simulink model "Robot_leg_3"  (R2018a)
settings: Solver=VariableStepAuto  StartTime=0.0  StopTime=10  RelTol=1e-3
model workspace: external: MATLAB File E:\Humanoid\Simscape model\Simscape_model_2\simscape_model\Robot_leg_2_DataFile.m (data not in the file)
values from neighbouring files (symbols this model uses):
  m = 0    [Trajectory_generation_initial.m]    (also in final_gait.m)
undefined symbols (not defined in the file or in its folder): height_plane, smiData, X, Y, Z
libraries: sm_lib x69, nesl_utility x52, simulink x49, walkingRobotUtils x14, Contact_Forces_Lib x8
(part 1 of 3)
settings Model: SimulationMode=external  Creator=Workstation-1  LastModifiedBy=Workstation-1
settings GRTTargetCC: ExtMode=on
settings DiagnosticsConfigSet: SimMechanicsRigidlyBoundBlock=none

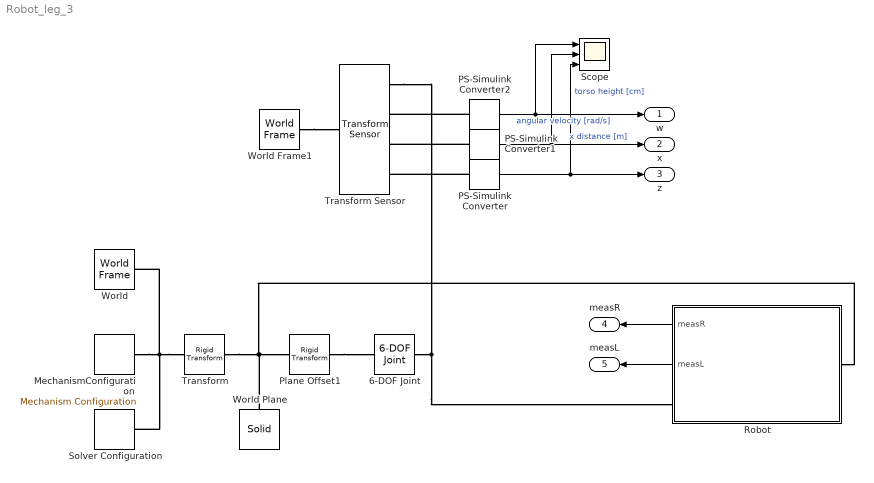
== system Robot_leg_3 ==
  6-DOF Joint : sm_lib/Joints/6-DOF Joint  SenseConstraintForce=off  SenseConstraintForceX=off  SenseConstraintForceY=off  SenseConstraintForceZ=off  SenseConstraintTorque=off  SenseConstraintTorqueX=off  SenseConstraintTorqueY=off  SenseConstraintTorqueZ=off  SenseTotalForce=off  SenseTotalForceX=off  SenseTotalForceY=off  SenseTotalForceZ=off  SenseTotalTorque=off  SenseTotalTorqueX=off  SenseTotalTorqueY=off  SenseTotalTorqueZ=off  CompositeWrenchDir=FollowerOnBase  CompositeWrenchFrame=BaseFrame  PxEquilibriumPosition=0  PxEquilibriumPositionUnits=m  PxSpringStiffness=0  PxSpringStiffnessUnits=N/m  PxDampingCoefficient=world_damping  PxDampingCoefficientUnits=N/(m/s)  PxTorqueActuationMode=NoTorque  PxMotionActuationMode=ComputedMotion  PxSensePosition=off  PxSenseVelocity=off  PxSenseAcceleration=off  PxSenseTorqueForce=off  PxPositionTargetSpecify=on  PxPositionTargetPriority=High  PxPositionTargetValue=0  PxPositionTargetValueUnits=m  PxVelocityTargetSpecify=off  PxVelocityTargetPriority=High  PxVelocityTargetValue=0  PxVelocityTargetValueUnits=m/s  PyEquilibriumPosition=0  PyEquilibriumPositionUnits=m  PySpringStiffness=0  PySpringStiffnessUnits=N/m  PyDampingCoefficient=world_damping  PyDampingCoefficientUnits=N/(m/s)  PyTorqueActuationMode=NoTorque  PyMotionActuationMode=ComputedMotion  PySensePosition=off  PySenseVelocity=off  PySenseAcceleration=off  PySenseTorqueForce=off  PyPositionTargetSpecify=on  PyPositionTargetPriority=High  PyPositionTargetValue=0  PyPositionTargetValueUnits=m  PyVelocityTargetSpecify=off  PyVelocityTargetPriority=High  PyVelocityTargetValue=0  PyVelocityTargetValueUnits=m/s  PzEquilibriumPosition=0  PzEquilibriumPositionUnits=m  PzSpringStiffness=0  PzSpringStiffnessUnits=N/m  PzDampingCoefficient=world_damping  PzDampingCoefficientUnits=N/(m/s)  PzTorqueActuationMode=NoTorque  PzMotionActuationMode=ComputedMotion  PzSensePosition=off  PzSenseVelocity=off  PzSenseAcceleration=off  PzSenseTorqueForce=off  PzPositionTargetSpecify=on  PzPositionTargetPriority=High  PzPositionTargetValue=init_height  PzPositionTargetValueUnits=cm  PzVelocityTargetSpecify=off  PzVelocityTargetPriority=High  PzVelocityTargetValue=0  PzVelocityTargetValueUnits=m/s  SphDefPosRotationMethod=None  SphDefPosRotationAngleUnits=deg  SphDefPosRotationStandardAxis=+Z  SphDefPosRotationAngle=0.0  SphDefPosRotationArbitraryAxis=[0 0 1]  SphDefPosFollAlignAxisA=+X  SphDefPosBaseAlignAxisA=+Y  SphDefPosFollAlignAxisB=+Y  SphDefPosBaseAlignAxisB=+Z  SphDefPosRotationSequenceAxes=FollowerAxes  SphDefPosRotationSequence=XYX  SphDefPosRotationSequenceAngles=[0 0 0]  SphDefPosRotationSequenceAnglesUnits=deg  SphDefPosRotationMatrix=[1 0 0; 0 1 0; 0 0 1]  SphEqPosRotationMethod=None  SphEqPosRotationAngleUnits=deg  SphEqPosRotationStandardAxis=+Z  SphEqPosRotationAngle=0.0  SphEqPosRotationArbitraryAxis=[0 0 1]  SphEqPosFollAlignAxisA=+X  SphEqPosBaseAlignAxisA=+Y  SphEqPosFollAlignAxisB=+Y  SphEqPosBaseAlignAxisB=+Z  SphEqPosRotationSequenceAxes=FollowerAxes  SphEqPosRotationSequence=XYX  SphEqPosRotationSequenceAngles=[0 0 0]  SphEqPosRotationSequenceAnglesUnits=deg  SphEqPosRotationMatrix=[1 0 0; 0 1 0; 0 0 1]  SphSpringStiffness=0  SphSpringStiffnessUnits=N*m/deg  SphDampingCoefficient=world_rot_damping  SphDampingCoefficientUnits=N*m/(rad/s)  SphActuateTorqueX=off  SphActuateTorqueY=off  SphActuateTorqueZ=off  SphActuateTorque=off  SphTorqueActuationMode=NoTorque  SphMotionActuationMode=ComputedMotion  SphActuationFrame=BaseFrame  SphSensePosition=off  SphSenseVelocityX=off  SphSenseVelocityY=off  SphSenseVelocityZ=off  SphSenseVelocity=off  SphSenseAccelerationX=off  SphSenseAccelerationY=off  SphSenseAccelerationZ=off  SphSenseAcceleration=off  SphSenseTorqueX=off  SphSenseTorqueY=off  SphSenseTorqueZ=off  SphSenseTorqueForce=off  SphSensingFrame=BaseFrame  SphPositionTargetRotationMethod=None  SphPositionTargetRotationAngleUnits=deg  SphPositionTargetRotationStandardAxis=+Z  SphPositionTargetRotationAngle=0.0  SphPositionTargetRotationArbitraryAxis=[0 0 1]  SphPositionTargetFollAlignAxisA=+X  SphPositionTargetBaseAlignAxisA=+Y  SphPositionTargetFollAlignAxisB=+Y  SphPositionTargetBaseAlignAxisB=+Z  SphPositionTargetRotationSequenceAxes=FollowerAxes  SphPositionTargetRotationSequence=XYX  SphPositionTargetRotationSequenceAngles=[0 0 0]  SphPositionTargetRotationSequenceAnglesUnits=deg  SphPositionTargetRotationMatrix=eye(3)  SphPositionTargetSpecify=off  SphPositionTargetPriority=High  SphVelocityTargetValue=[0 0 0]  SphVelocityTargetValueUnits=deg/s  SphVelocityTargetSpecify=off  SphVelocityTargetPriority=High  SphVelocityTargetInFollowerFrame=on
  MechanismConfiguration : sm_lib/Utilities/Mechanism Configuration  UniformGravity=Constant  GravityVector=[0 0 -9.80665]  GravityUnits=m/s^2  LinearizationDelta=0.001
  PS-Simulink Converter : nesl_utility/PS-Simulink Converter  PhysicalDomain=network_engine_domain  SubClassName=ps_output  LeftPortType=input  RightPortType=output  PseudoPeriodic=off  Frequencies=[]  Unit=cm  AffineConversion=off
  PS-Simulink Converter1 : nesl_utility/PS-Simulink Converter  PhysicalDomain=network_engine_domain  SubClassName=ps_output  LeftPortType=input  RightPortType=output  PseudoPeriodic=off  Frequencies=[]  Unit=m  AffineConversion=off
  PS-Simulink Converter2 : nesl_utility/PS-Simulink Converter  PhysicalDomain=network_engine_domain  SubClassName=ps_output  LeftPortType=input  RightPortType=output  PseudoPeriodic=off  Frequencies=[]  Unit=rad/s  AffineConversion=off
  Plane Offset1 : sm_lib/Frames and Transforms/Rigid Transform  TranslationMethod=StandardAxis  TranslationStandardOffset=height_plane/2  TranslationLengthUnit=m  TranslationStandardAxis=+Z  TranslationCartesianOffset=[0 0 0]  TranslationROffset=0  TranslationROffsetUnits=m  TranslationZOffset=0  TranslationZOffsetUnits=m  TranslationThetaOffset=0  TranslationThetaOffsetUnits=deg  RotationMethod=None  RotationAngleUnits=deg  RotationStandardAxis=+Z  RotationAngle=0.0  RotationArbitraryAxis=[0 0 1]  FollAlignAxisA=+X  BaseAlignAxisA=+Y  FollAlignAxisB=+Y  BaseAlignAxisB=+Z  RotationSequenceAxes=FollowerAxes  RotationSequence=XYX  RotationSequenceAngles=[0 0 0]  RotationSequenceAnglesUnits=deg  RotationMatrix=[1 0 0; 0 1 0; 0 0 1]
  Robot : Subsystem
  Scope : Scope  NumInputPorts=3
  Solver Configuration : nesl_utility/Solver Configuration  PhysicalDomain=network_engine_domain  SubClassName=solver  LeftPortType=input  RightPortType=generic  Tones=[]  Harmonics=[]  SimulateNoise=off  Profile=off  UseLocalSampling=off  EnableSwitchedLinearOptims=on  FrequencyDomain=off  UseCCode=off  RelTol=0.001  AbsTol=1e-06  MinStep=1e-09  ToWorkspace=off  RevertToSquareIcSolve=off  NumHomotopyIterations=100  PhasorMode=off  PhasorModeNumHarmonics=1  DoDC=off  ResidualTolerance=1e-09  UseLocalSolver=off  LocalSolverChoice=NE_BACKWARD_EULER_ADVANCER  LocalSolverSampleTime=0.001  DoFixedCost=off  MaxNonlinIter=3  MaxModeIter=2  LinearAlgebra=Sparse  EquationFormulation=NE_TIME_EF  DelaysMemoryBudget=1024  AutomaticFiltering=on  FilteringTimeConstant=0.001
  Transform : sm_lib/Frames and Transforms/Rigid Transform  TranslationMethod=Cartesian  TranslationStandardOffset=0  TranslationLengthUnit=mm  TranslationStandardAxis=+Z  TranslationCartesianOffset=smiData.RigidTransform(22).translation  TranslationROffset=0  TranslationROffsetUnits=m  TranslationZOffset=0  TranslationZOffsetUnits=m  TranslationThetaOffset=0  TranslationThetaOffsetUnits=deg  RotationMethod=ArbitraryAxis  RotationAngleUnits=rad  RotationStandardAxis=+Z  RotationAngle=smiData.RigidTransform(22).angle  RotationArbitraryAxis=smiData.RigidTransform(22).axis  FollAlignAxisA=+X  BaseAlignAxisA=+Y  FollAlignAxisB=+Y  BaseAlignAxisB=+Z  RotationSequenceAxes=FollowerAxes  RotationSequence=XYX  RotationSequenceAngles=[0 0 0]  RotationSequenceAnglesUnits=deg  RotationMatrix=[1 0 0; 0 1 0; 0 0 1]
  Transform Sensor : sm_lib/Frames and Transforms/Transform Sensor  MeasurementFrame=World  SenseAngle=off  SenseAxis=off  SenseAngle1=off  SenseAngle2=off  SenseAngle3=off  SenseQ=off  SenseR=off  SenseOmegaX=off  SenseOmegaY=off  SenseOmegaZ=on  SenseOmega1=off  SenseOmega2=off  SenseOmega3=off  SenseQDot=off  SenseRDot=off  SenseAlphaX=off  SenseAlphaY=off  SenseAlphaZ=off  SenseAlpha1=off  SenseAlpha2=off  SenseAlpha3=off  SenseQDDot=off  SenseRDDot=off  SenseX=on  SenseY=off  SenseZ=on  SenseRad=off  SenseAzim=off  SenseDist=off  SenseInc=off  SenseXDot=off  SenseYDot=off  SenseZDot=off  SenseRadDot=off  SenseAzimDot=off  SenseDistDot=off  SenseIncDot=off  SenseXDDot=off  SenseYDDot=off  SenseZDDot=off  SenseRadDDot=off  SenseAzimDDot=off  SenseDistDDot=off  SenseIncDDot=off
  World : sm_lib/Frames and Transforms/World Frame
  World Frame1 : sm_lib/Frames and Transforms/World Frame
  World Plane : sm_lib/Body Elements/Solid  InertiaType=CalculateFromGeometry  Mass=1  MassUnits=kg  CenterOfMass=[0 0 0]  CenterOfMassUnits=m  MomentsOfInertia=[1 1 1]  MomentsOfInertiaUnits=kg*m^2  ProductsOfInertia=[0 0 0]  ProductsOfInertiaUnits=kg*m^2  DensityBased=on  Density=density  DensityUnits=kg/(m^3)  DoExposeReferenceFrame=on  SerializedFrames=<Frames/>  GraphicType=FromGeometry  MarkerShape=Sphere  MarkerSize=10  MarkerSizeUnits=m  GraphicVisPropType=SimpleVisualProperties  GraphicDiffuseColor=[1.0 1.0 0.8]  GraphicSpecularColor=[0.5 0.5 0.5 1.0]  GraphicAmbientColor=[0.15 0.15 0.15 1.0]  GraphicEmissiveColor=[0.0 0.0 0.0 1.0]  GraphicShininess=75  GraphicOpacity=0.5  GeometryShape=Brick  RectangleSize=[1 1]  RectangleSizeUnits=m  BrickDimensions="[10 3  0.025]"  BrickDimensionUnits=m  CylinderRadius=1  CylinderRadiusUnits=m  CylinderLength=1  CylinderLengthUnits=m  SphereRadius=1  SphereRadiusUnits=m  EllipsoidRadii=[1 1 1]  EllipsoidRadiiUnits=m  ExtrusionCrossSection=[1 1; -1 1; -1 -1; 1 -1]  ExtrusionCrossSectionUnits=m  ExtrusionLength=1  ExtrusionLengthUnits=m  PolygonNumSides=3  PolygonOuterRadius=1  PolygonOuterRadiusUnits=m  ExtGeomFileType=STL  ExtGeomFileUnits=m  RevolutionCrossSection=[1 1; 1 -1; 2 -1; 2 1]  RevolutionCrossSectionUnits=m  RevolutionExtent=Full  RevolutionAngle=180  RevolutionAngleUnits=deg
  w : Outport
  x : Outport  Port=2
  z : Outport  Port=3
  measR : Outport  Port=4
  measL : Outport  Port=5
  wires:
  PS-Simulink Converter/1 -> Scope/3, z/1  "torso height [cm]"
  PS-Simulink Converter2/1 -> Scope/1, w/1  "angular velocity [rad/s]"
  PS-Simulink Converter1/1 -> Scope/2, x/1  "x distance [m]"
  Robot/1(measR) -> measR/1
  Robot/2(measL) -> measL/1
  connections:
  Transform/LConn1 -- Solver Configuration/RConn1 -- MechanismConfiguration/RConn1 -- World/RConn1
  Transform/RConn1 -- Plane Offset1/LConn1 -- World Plane/RConn1 -- Robot/LConn1
  6-DOF Joint/RConn1 -- Robot/RConn1 -- Transform Sensor/RConn1
  Plane Offset1/RConn1 -- 6-DOF Joint/LConn1
  PS-Simulink Converter1/LConn1 -- Transform Sensor/RConn3
  PS-Simulink Converter/LConn1 -- Transform Sensor/RConn4
  PS-Simulink Converter2/LConn1 -- Transform Sensor/RConn2
  World Frame1/RConn1 -- Transform Sensor/LConn1

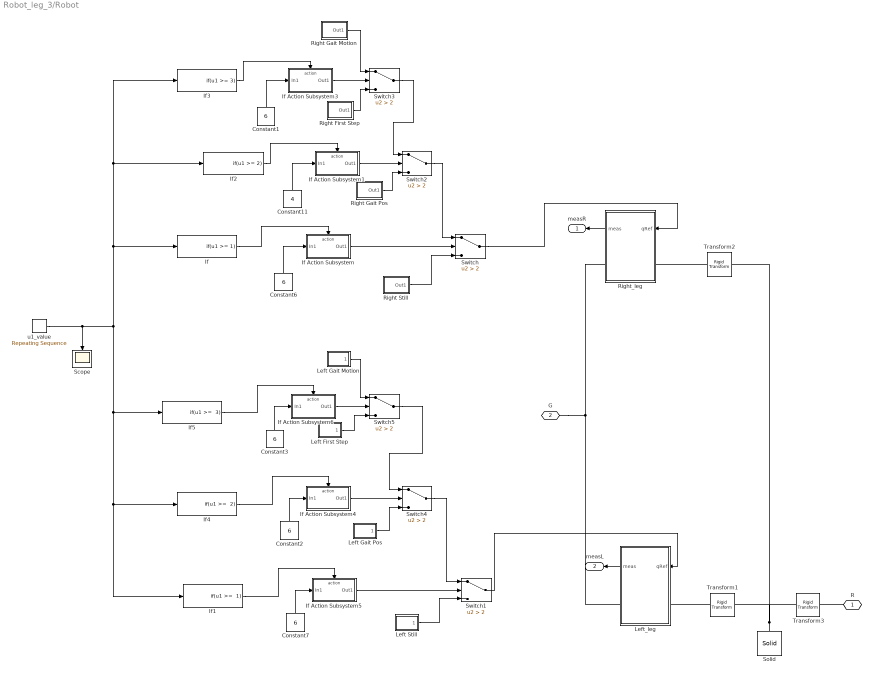
== system Robot_leg_3/Robot ==
  Constant{1..3,6..7} (5 alike) : Constant  Value=6
  Constant11 : Constant  Value=4
  If : If  IfExpression=u1 >= 1  ShowElse=off
  If Action Subsystem : Subsystem  TreatAsAtomicUnit=on
  If Action Subsystem1 : Subsystem  TreatAsAtomicUnit=on
  If Action Subsystem3 : Subsystem  TreatAsAtomicUnit=on
  If Action Subsystem4 : Subsystem  TreatAsAtomicUnit=on
  If Action Subsystem5 : Subsystem  TreatAsAtomicUnit=on
  If Action Subsystem6 : Subsystem  TreatAsAtomicUnit=on
  If1 : If  IfExpression="u1 >=  1"  ShowElse=off
  If2 : If  IfExpression=u1 >= 2  ShowElse=off
  If3 : If  IfExpression=u1 >= 3  ShowElse=off
  If4 : If  IfExpression="u1 >=  2"  ShowElse=off
  If5 : If  IfExpression="u1 >=  3"  ShowElse=off
  Left First Step : Subsystem
  Left Gait Motion : Subsystem
  Left Gait Pos : Subsystem
  Left Still : Subsystem
  Left_leg : Subsystem
  Right First Step : Subsystem
  Right Gait Motion : Subsystem
  Right Gait Pos : Subsystem
  Right Still : Subsystem
  Right_leg : Subsystem
  Scope : Scope
  Solid : sm_lib/Body Elements/Solid  InertiaType=Custom  Mass=smiData.Solid(13).mass  MassUnits=kg  CenterOfMass=smiData.Solid(13).CoM  CenterOfMassUnits=mm  MomentsOfInertia=smiData.Solid(13).MoI  MomentsOfInertiaUnits=kg*mm^2  ProductsOfInertia=smiData.Solid(13).PoI  ProductsOfInertiaUnits=kg*mm^2  DensityBased=on  Density=1000  DensityUnits=kg/m^3  DoExposeReferenceFrame=on  SerializedFrames=<Frames/>  GraphicType=FromGeometry  MarkerShape=Sphere  MarkerSize=10  GraphicVisPropType=SimpleVisualProperties  GraphicDiffuseColor=smiData.Solid(13).color  GraphicSpecularColor=[0.5 0.5 0.5 1.0]  GraphicAmbientColor=[0.15 0.15 0.15 1.0]  GraphicEmissiveColor=[0.0 0.0 0.0 1.0]  GraphicShininess=75  GraphicOpacity=smiData.Solid(13).opacity  GeometryShape=FromFile  RectangleSize=[1 1]  RectangleSizeUnits=m  BrickDimensions=[1 1 1]  BrickDimensionUnits=m  CylinderRadius=1  CylinderRadiusUnits=m  CylinderLength=1  CylinderLengthUnits=m  SphereRadius=1  SphereRadiusUnits=m  EllipsoidRadii=[1 1 1]  EllipsoidRadiiUnits=m  ExtrusionCrossSection=[1 1; -1 1; -1 -1; 1 -1]  ExtrusionCrossSectionUnits=m  ExtrusionLength=1  ExtrusionLengthUnits=m  PolygonNumSides=3  PolygonOuterRadius=1  PolygonOuterRadiusUnits=m  ExtGeomFileType=STEP  ExtGeomFileName=Torso_Default_sldprt.STEP  ExtGeomFileUnits=m  RevolutionCrossSection=[1 1; 1 -1; 2 -1; 2 1]  RevolutionCrossSectionUnits=m  RevolutionExtent=Full  RevolutionAngle=180  RevolutionAngleUnits=deg
  Switch{,1..5} (6 alike) : Switch  Criteria=u2 > Threshold  Threshold=2
  Transform1 : sm_lib/Frames and Transforms/Rigid Transform  TranslationMethod=Cartesian  TranslationStandardOffset=0  TranslationLengthUnit=mm  TranslationStandardAxis=+Z  TranslationCartesianOffset=smiData.RigidTransform(17).translation  TranslationROffset=0  TranslationROffsetUnits=m  TranslationZOffset=0  TranslationZOffsetUnits=m  TranslationThetaOffset=0  TranslationThetaOffsetUnits=deg  RotationMethod=ArbitraryAxis  RotationAngleUnits=rad  RotationStandardAxis=+Z  RotationAngle=smiData.RigidTransform(17).angle  RotationArbitraryAxis=smiData.RigidTransform(17).axis  FollAlignAxisA=+X  BaseAlignAxisA=+Y  FollAlignAxisB=+Y  BaseAlignAxisB=+Z  RotationSequenceAxes=FollowerAxes  RotationSequence=XYX  RotationSequenceAngles=[0 0 0]  RotationSequenceAnglesUnits=deg  RotationMatrix=[1 0 0; 0 1 0; 0 0 1]
  Transform2 : sm_lib/Frames and Transforms/Rigid Transform  TranslationMethod=Cartesian  TranslationStandardOffset=0  TranslationLengthUnit=mm  TranslationStandardAxis=+Z  TranslationCartesianOffset=smiData.RigidTransform(19).translation  TranslationROffset=0  TranslationROffsetUnits=m  TranslationZOffset=0  TranslationZOffsetUnits=m  TranslationThetaOffset=0  TranslationThetaOffsetUnits=deg  RotationMethod=ArbitraryAxis  RotationAngleUnits=rad  RotationStandardAxis=+Z  RotationAngle=smiData.RigidTransform(19).angle  RotationArbitraryAxis=smiData.RigidTransform(19).axis  FollAlignAxisA=+X  BaseAlignAxisA=+Y  FollAlignAxisB=+Y  BaseAlignAxisB=+Z  RotationSequenceAxes=FollowerAxes  RotationSequence=XYX  RotationSequenceAngles=[0 0 0]  RotationSequenceAnglesUnits=deg  RotationMatrix=[1 0 0; 0 1 0; 0 0 1]
  Transform3 : sm_lib/Frames and Transforms/Rigid Transform  TranslationMethod=Cartesian  TranslationStandardOffset=0  TranslationLengthUnit=mm  TranslationStandardAxis=+Z  TranslationCartesianOffset=smiData.RigidTransform(21).translation  TranslationROffset=0  TranslationROffsetUnits=m  TranslationZOffset=0  TranslationZOffsetUnits=m  TranslationThetaOffset=0  TranslationThetaOffsetUnits=deg  RotationMethod=ArbitraryAxis  RotationAngleUnits=rad  RotationStandardAxis=+Z  RotationAngle=smiData.RigidTransform(21).angle  RotationArbitraryAxis=smiData.RigidTransform(21).axis  FollAlignAxisA=+X  BaseAlignAxisA=+Y  FollAlignAxisB=+Y  BaseAlignAxisB=+Z  RotationSequenceAxes=FollowerAxes  RotationSequence=XYX  RotationSequenceAngles=[0 0 0]  RotationSequenceAnglesUnits=deg  RotationMatrix=[1 0 0; 0 1 0; 0 0 1]
  "u1_value " : simulink/Sources/Repeating Sequence  rep_seq_t=total_time  rep_seq_y=u1
  R : PMIOPort  Side=Right
  G : PMIOPort  Port=2  Side=Left
  measR : Outport
  measL : Outport  Port=2
  wires:
  "u1_value "/1 -> Scope/1, If5/1, If4/1, If1/1, If2/1, If3/1, If/1
  Switch2/1 -> Switch/1
  If1/1 -> If Action Subsystem5/Action
  Constant1/1 -> If Action Subsystem3/1(In1)
  Switch5/1 -> Switch4/1
  If/1 -> If Action Subsystem/Action
  Constant6/1 -> If Action Subsystem/1(In1)
  If Action Subsystem/1(Out1) -> Switch/2
  If Action Subsystem6/1(Out1) -> Switch5/2
  Constant7/1 -> If Action Subsystem5/1(In1)
  Constant2/1 -> If Action Subsystem4/1(In1)
  If5/1 -> If Action Subsystem6/Action
  If4/1 -> If Action Subsystem4/Action
  If Action Subsystem3/1(Out1) -> Switch3/2
  If Action Subsystem5/1(Out1) -> Switch1/2
  Switch4/1 -> Switch1/1
  Constant3/1 -> If Action Subsystem6/1(In1)
  Switch1/1 -> Left_leg/1(qRef)
  If3/1 -> If Action Subsystem3/Action
  If Action Subsystem1/1(Out1) -> Switch2/2
  Right Still/1(Out1) -> Switch/3
  Left Still/1(Out1) -> Switch1/3
  Switch3/1 -> Switch2/1
  Switch/1 -> Right_leg/1(qRef)
  If Action Subsystem4/1(Out1) -> Switch4/2
  If2/1 -> If Action Subsystem1/Action
  Constant11/1 -> If Action Subsystem1/1(In1)
  Right Gait Motion/1(Out1) -> Switch3/1
  Left Gait Motion/1(Out1) -> Switch5/1
  Left Gait Pos/1(Out1) -> Switch4/3
  Left First Step/1(Out1) -> Switch5/3
  Right First Step/1(Out1) -> Switch3/3
  Right Gait Pos/1(Out1) -> Switch2/3
  Left_leg/1(meas) -> measL/1
  Right_leg/1(meas) -> measR/1
  connections:
  Solid/RConn1 -- Transform2/LConn1 -- Transform1/LConn1 -- Transform3/LConn1
  R/RConn1 -- Transform3/RConn1
  Transform2/RConn1 -- Right_leg/LConn1
  Transform1/RConn1 -- Left_leg/LConn1
  Left_leg/RConn1 -- G/RConn1 -- Right_leg/RConn1

== system Robot_leg_3/Robot/If Action Subsystem ==
  In1 : Inport
  Action Port : ActionPort  ActionType=then
  Out1 : Outport
  wires:
  In1/1 -> Out1/1

== system Robot_leg_3/Robot/If Action Subsystem1 ==
  In1 : Inport
  Action Port : ActionPort  ActionType=then
  Out1 : Outport
  wires:
  In1/1 -> Out1/1

== system Robot_leg_3/Robot/If Action Subsystem3 ==
  In1 : Inport
  Action Port : ActionPort  ActionType=then
  Out1 : Outport
  wires:
  In1/1 -> Out1/1

== system Robot_leg_3/Robot/If Action Subsystem4 ==
  In1 : Inport
  Action Port : ActionPort  ActionType=then
  Out1 : Outport
  wires:
  In1/1 -> Out1/1

== system Robot_leg_3/Robot/If Action Subsystem5 ==
  In1 : Inport
  Action Port : ActionPort  ActionType=then
  Out1 : Outport
  wires:
  In1/1 -> Out1/1

== system Robot_leg_3/Robot/If Action Subsystem6 ==
  In1 : Inport
  Action Port : ActionPort  ActionType=then
  Out1 : Outport
  wires:
  In1/1 -> Out1/1

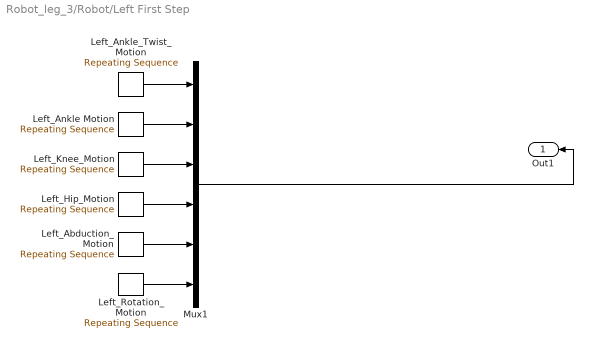
== system Robot_leg_3/Robot/Left First Step ==
  Left_Abduction_Motion : simulink/Sources/Repeating Sequence  rep_seq_t=time  rep_seq_y=left_theta_first_5
  Left_Ankle Motion : simulink/Sources/Repeating Sequence  rep_seq_t=time_first  rep_seq_y=left_theta_first_3
  Left_Ankle_Twist_Motion : simulink/Sources/Repeating Sequence  rep_seq_t=time  rep_seq_y=left_theta_first_4
  Left_Hip_Motion : simulink/Sources/Repeating Sequence  rep_seq_t=time_first  rep_seq_y=left_theta_first_1
  Left_Knee_Motion : simulink/Sources/Repeating Sequence  rep_seq_t=time_first  rep_seq_y=left_theta_first_2
  Left_Rotation_Motion : simulink/Sources/Repeating Sequence  rep_seq_t=time_first  rep_seq_y=left_theta_first_6
  Mux1 : Mux  Inputs=6
  Out1 : Outport
  wires:
  Left_Knee_Motion/1 -> Mux1/3
  Left_Rotation_Motion/1 -> Mux1/6
  Left_Hip_Motion/1 -> Mux1/4
  Left_Abduction_Motion/1 -> Mux1/5
  Left_Ankle_Twist_Motion/1 -> Mux1/1
  Left_Ankle Motion/1 -> Mux1/2
  Mux1/1 -> Out1/1

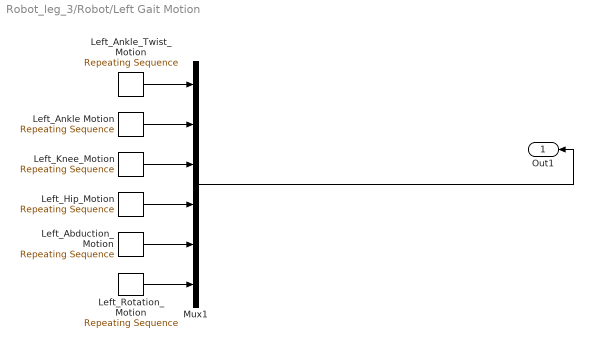
== system Robot_leg_3/Robot/Left Gait Motion ==
  Left_Abduction_Motion : simulink/Sources/Repeating Sequence  rep_seq_t=time  rep_seq_y=left_theta_5
  Left_Ankle Motion : simulink/Sources/Repeating Sequence  rep_seq_t=time  rep_seq_y=left_theta_3
  Left_Ankle_Twist_Motion : simulink/Sources/Repeating Sequence  rep_seq_t=time  rep_seq_y=left_theta_4
  Left_Hip_Motion : simulink/Sources/Repeating Sequence  rep_seq_t=time  rep_seq_y=left_theta_1
  Left_Knee_Motion : simulink/Sources/Repeating Sequence  rep_seq_t=time  rep_seq_y=left_theta_2
  Left_Rotation_Motion : simulink/Sources/Repeating Sequence  rep_seq_t=time  rep_seq_y=left_theta_6
  Mux1 : Mux  Inputs=6
  Out1 : Outport
  wires:
  Left_Knee_Motion/1 -> Mux1/3
  Left_Rotation_Motion/1 -> Mux1/6
  Left_Hip_Motion/1 -> Mux1/4
  Left_Abduction_Motion/1 -> Mux1/5
  Left_Ankle_Twist_Motion/1 -> Mux1/1
  Left_Ankle Motion/1 -> Mux1/2
  Mux1/1 -> Out1/1

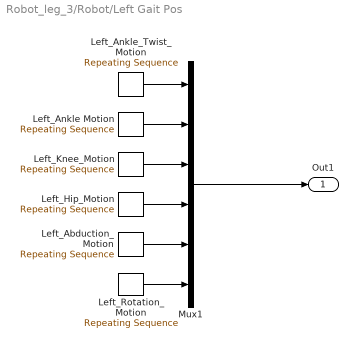
== system Robot_leg_3/Robot/Left Gait Pos ==
  Left_Abduction_Motion : simulink/Sources/Repeating Sequence  rep_seq_t=time  rep_seq_y=left_theta_pos_5
  Left_Ankle Motion : simulink/Sources/Repeating Sequence  rep_seq_t=time  rep_seq_y=left_theta_pos_3
  Left_Ankle_Twist_Motion : simulink/Sources/Repeating Sequence  rep_seq_t=time  rep_seq_y=left_theta_pos_4
  Left_Hip_Motion : simulink/Sources/Repeating Sequence  rep_seq_t=time  rep_seq_y=left_theta_pos_1
  Left_Knee_Motion : simulink/Sources/Repeating Sequence  rep_seq_t=time  rep_seq_y=left_theta_pos_2
  Left_Rotation_Motion : simulink/Sources/Repeating Sequence  rep_seq_t=time  rep_seq_y=left_theta_pos_6
  Mux1 : Mux  Inputs=6
  Out1 : Outport
  wires:
  Mux1/1 -> Out1/1
  Left_Ankle Motion/1 -> Mux1/2
  Left_Ankle_Twist_Motion/1 -> Mux1/1
  Left_Abduction_Motion/1 -> Mux1/5
  Left_Hip_Motion/1 -> Mux1/4
  Left_Rotation_Motion/1 -> Mux1/6
  Left_Knee_Motion/1 -> Mux1/3

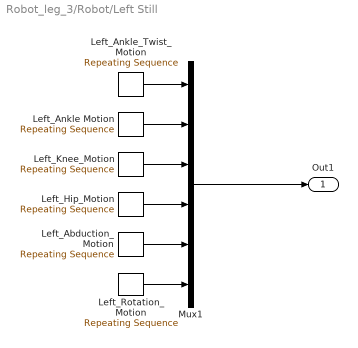
== system Robot_leg_3/Robot/Left Still ==
  Left_Abduction_Motion : simulink/Sources/Repeating Sequence  rep_seq_t=time  rep_seq_y=left_theta_init_5
  Left_Ankle Motion : simulink/Sources/Repeating Sequence  rep_seq_t=time  rep_seq_y=left_theta_init_3
  Left_Ankle_Twist_Motion : simulink/Sources/Repeating Sequence  rep_seq_t=time  rep_seq_y=left_theta_init_4
  Left_Hip_Motion : simulink/Sources/Repeating Sequence  rep_seq_t=time  rep_seq_y=left_theta_init_1
  Left_Knee_Motion : simulink/Sources/Repeating Sequence  rep_seq_t=time  rep_seq_y=left_theta_init_2
  Left_Rotation_Motion : simulink/Sources/Repeating Sequence  rep_seq_t=time  rep_seq_y=left_theta_init_6
  Mux1 : Mux  Inputs=6
  Out1 : Outport
  wires:
  Mux1/1 -> Out1/1
  Left_Ankle Motion/1 -> Mux1/2
  Left_Ankle_Twist_Motion/1 -> Mux1/1
  Left_Abduction_Motion/1 -> Mux1/5
  Left_Hip_Motion/1 -> Mux1/4
  Left_Rotation_Motion/1 -> Mux1/6
  Left_Knee_Motion/1 -> Mux1/3

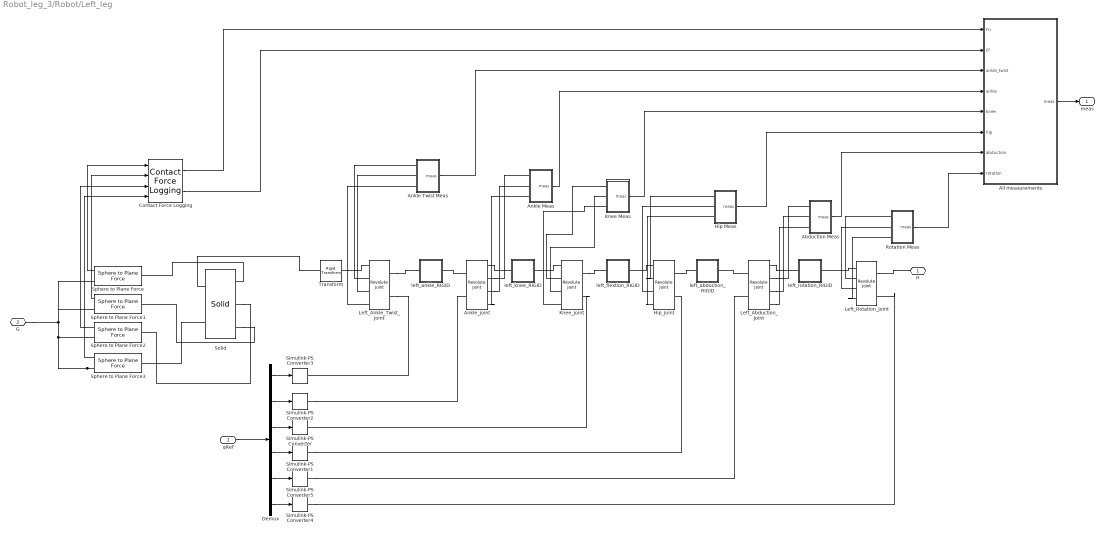
== system Robot_leg_3/Robot/Left_leg ==
  qRef : Inport
  Abduction Meas : Subsystem
  All measurements : Subsystem
  Ankle Meas : Subsystem
  Ankle Twist Meas : Subsystem
  Ankle_joint : sm_lib/Joints/Revolute Joint  SenseConstraintForce=off  SenseConstraintForceX=off  SenseConstraintForceY=off  SenseConstraintForceZ=off  SenseConstraintTorque=off  SenseConstraintTorqueX=off  SenseConstraintTorqueY=off  SenseConstraintTorqueZ=off  SenseTotalForce=off  SenseTotalForceX=off  SenseTotalForceY=off  SenseTotalForceZ=off  SenseTotalTorque=off  SenseTotalTorqueX=off  SenseTotalTorqueY=off  SenseTotalTorqueZ=off  CompositeWrenchDir=FollowerOnBase  CompositeWrenchFrame=BaseFrame  EquilibriumPosition=0  EquilibriumPositionUnits=rad  SpringStiffness=0  SpringStiffnessUnits=N*m/rad  DampingCoefficient=0  DampingCoefficientUnits=N*m/(rad/s)  TorqueActuationMode=ComputedTorque  MotionActuationMode=InputMotion  SensePosition=on  SenseVelocity=on  SenseAcceleration=off  SenseTorqueForce=on  PositionTargetSpecify=on  PositionTargetPriority=Low  PositionTargetValue=smiData.RevoluteJoint(7).Rz.Pos  PositionTargetValueUnits=deg  VelocityTargetSpecify=off  VelocityTargetPriority=High  VelocityTargetValue=0  VelocityTargetValueUnits=deg/s
  Contact Force Logging : walkingRobotUtils/Contact Force Logging
  Demux : Demux  Outputs=6
  Hip Meas : Subsystem
  Hip_Joint : sm_lib/Joints/Revolute Joint  SenseConstraintForce=off  SenseConstraintForceX=off  SenseConstraintForceY=off  SenseConstraintForceZ=off  SenseConstraintTorque=off  SenseConstraintTorqueX=off  SenseConstraintTorqueY=off  SenseConstraintTorqueZ=off  SenseTotalForce=off  SenseTotalForceX=off  SenseTotalForceY=off  SenseTotalForceZ=off  SenseTotalTorque=off  SenseTotalTorqueX=off  SenseTotalTorqueY=off  SenseTotalTorqueZ=off  CompositeWrenchDir=FollowerOnBase  CompositeWrenchFrame=BaseFrame  EquilibriumPosition=0  EquilibriumPositionUnits=rad  SpringStiffness=0  SpringStiffnessUnits=N*m/rad  DampingCoefficient=0  DampingCoefficientUnits=N*m/(rad/s)  TorqueActuationMode=ComputedTorque  MotionActuationMode=InputMotion  SensePosition=on  SenseVelocity=on  SenseAcceleration=off  SenseTorqueForce=on  PositionTargetSpecify=on  PositionTargetPriority=Low  PositionTargetValue=smiData.RevoluteJoint(12).Rz.Pos  PositionTargetValueUnits=deg  VelocityTargetSpecify=off  VelocityTargetPriority=High  VelocityTargetValue=0  VelocityTargetValueUnits=deg/s
  Knee Meas : Subsystem
  Knee_joint : sm_lib/Joints/Revolute Joint  SenseConstraintForce=off  SenseConstraintForceX=off  SenseConstraintForceY=off  SenseConstraintForceZ=off  SenseConstraintTorque=off  SenseConstraintTorqueX=off  SenseConstraintTorqueY=off  SenseConstraintTorqueZ=off  SenseTotalForce=off  SenseTotalForceX=off  SenseTotalForceY=off  SenseTotalForceZ=off  SenseTotalTorque=off  SenseTotalTorqueX=off  SenseTotalTorqueY=off  SenseTotalTorqueZ=off  CompositeWrenchDir=FollowerOnBase  CompositeWrenchFrame=BaseFrame  EquilibriumPosition=0  EquilibriumPositionUnits=rad  SpringStiffness=0  SpringStiffnessUnits=N*m/rad  DampingCoefficient=0  DampingCoefficientUnits=N*m/(rad/s)  TorqueActuationMode=ComputedTorque  MotionActuationMode=InputMotion  SensePosition=on  SenseVelocity=on  SenseAcceleration=off  SenseTorqueForce=on  PositionTargetSpecify=on  PositionTargetPriority=Low  PositionTargetValue=smiData.RevoluteJoint(11).Rz.Pos  PositionTargetValueUnits=deg  VelocityTargetSpecify=off  VelocityTargetPriority=High  VelocityTargetValue=0  VelocityTargetValueUnits=deg/s
  Left_Abduction_Joint : sm_lib/Joints/Revolute Joint  SenseConstraintForce=off  SenseConstraintForceX=off  SenseConstraintForceY=off  SenseConstraintForceZ=off  SenseConstraintTorque=off  SenseConstraintTorqueX=off  SenseConstraintTorqueY=off  SenseConstraintTorqueZ=off  SenseTotalForce=off  SenseTotalForceX=off  SenseTotalForceY=off  SenseTotalForceZ=off  SenseTotalTorque=off  SenseTotalTorqueX=off  SenseTotalTorqueY=off  SenseTotalTorqueZ=off  CompositeWrenchDir=FollowerOnBase  CompositeWrenchFrame=BaseFrame  EquilibriumPosition=0  EquilibriumPositionUnits=rad  SpringStiffness=0  SpringStiffnessUnits=N*m/rad  DampingCoefficient=0  DampingCoefficientUnits=N*m/(rad/s)  TorqueActuationMode=ComputedTorque  MotionActuationMode=InputMotion  SensePosition=on  SenseVelocity=on  SenseAcceleration=off  SenseTorqueForce=on  PositionTargetSpecify=on  PositionTargetPriority=Low  PositionTargetValue=smiData.RevoluteJoint(4).Rz.Pos  PositionTargetValueUnits=deg  VelocityTargetSpecify=off  VelocityTargetPriority=High  VelocityTargetValue=0  VelocityTargetValueUnits=deg/s
  Left_Ankle_Twist_Joint : sm_lib/Joints/Revolute Joint  SenseConstraintForce=off  SenseConstraintForceX=off  SenseConstraintForceY=off  SenseConstraintForceZ=off  SenseConstraintTorque=off  SenseConstraintTorqueX=off  SenseConstraintTorqueY=off  SenseConstraintTorqueZ=off  SenseTotalForce=off  SenseTotalForceX=off  SenseTotalForceY=off  SenseTotalForceZ=off  SenseTotalTorque=off  SenseTotalTorqueX=off  SenseTotalTorqueY=off  SenseTotalTorqueZ=off  CompositeWrenchDir=FollowerOnBase  CompositeWrenchFrame=BaseFrame  EquilibriumPosition=0  EquilibriumPositionUnits=rad  SpringStiffness=0  SpringStiffnessUnits=N*m/rad  DampingCoefficient=0  DampingCoefficientUnits=N*m/(rad/s)  TorqueActuationMode=ComputedTorque  MotionActuationMode=InputMotion  SensePosition=on  SenseVelocity=on  SenseAcceleration=off  SenseTorqueForce=on  PositionTargetSpecify=on  PositionTargetPriority=Low  PositionTargetValue=smiData.RevoluteJoint(6).Rz.Pos  PositionTargetValueUnits=deg  VelocityTargetSpecify=off  VelocityTargetPriority=High  VelocityTargetValue=0  VelocityTargetValueUnits=deg/s
  Left_Rotation_Joint : sm_lib/Joints/Revolute Joint  SenseConstraintForce=off  SenseConstraintForceX=off  SenseConstraintForceY=off  SenseConstraintForceZ=off  SenseConstraintTorque=off  SenseConstraintTorqueX=off  SenseConstraintTorqueY=off  SenseConstraintTorqueZ=off  SenseTotalForce=off  SenseTotalForceX=off  SenseTotalForceY=off  SenseTotalForceZ=off  SenseTotalTorque=off  SenseTotalTorqueX=off  SenseTotalTorqueY=off  SenseTotalTorqueZ=off  CompositeWrenchDir=FollowerOnBase  CompositeWrenchFrame=BaseFrame  EquilibriumPosition=0  EquilibriumPositionUnits=rad  SpringStiffness=0  SpringStiffnessUnits=N*m/rad  DampingCoefficient=0  DampingCoefficientUnits=N*m/(rad/s)  TorqueActuationMode=ComputedTorque  MotionActuationMode=InputMotion  SensePosition=on  SenseVelocity=on  SenseAcceleration=off  SenseTorqueForce=on  PositionTargetSpecify=on  PositionTargetPriority=Low  PositionTargetValue=smiData.RevoluteJoint(9).Rz.Pos  PositionTargetValueUnits=deg  VelocityTargetSpecify=off  VelocityTargetPriority=High  VelocityTargetValue=0  VelocityTargetValueUnits=deg/s
  Rotation Meas : Subsystem
  Simulink-PS Converter{,1..5} (6 alike) : nesl_utility/Simulink-PS Converter  PhysicalDomain=network_engine_domain  SubClassName=ps_input  LeftPortType=input  RightPortType=output  PseudoPeriodic=off  Frequencies=[]  NoiseDistribution=none  NoiseParameters=[]  Unit=rad  AffineConversion=off  FilteringAndDerivatives=filter  SimscapeFilterOrder=2  InputFilterTimeConstant=motion_time_constant  UdotUserProvided=1
  Solid : sm_lib/Body Elements/Solid  InertiaType=Custom  Mass=smiData.Solid(10).mass  MassUnits=kg  CenterOfMass=smiData.Solid(10).CoM  CenterOfMassUnits=mm  MomentsOfInertia=smiData.Solid(10).MoI  MomentsOfInertiaUnits=kg*mm^2  ProductsOfInertia=smiData.Solid(10).PoI  ProductsOfInertiaUnits=kg*mm^2  DensityBased=on  Density=1000  DensityUnits=kg/m^3  DoExposeReferenceFrame=on  SerializedFrames=<Frames><Frame><Id>Frame1</Id><Value><Name>F1</Name><Origin><Source>GeometricFeature</Source><FeatureName>point 1082</FeatureName></Origin><PrimaryAxis><DefinedDirection>+Z</DefinedDirection><Source>ReferenceFrame</Source><SourceDirection>+Z</SourceDirection><FeatureName></FeatureName></PrimaryAxis><SecondaryAxis><DefinedDirection>+X</DefinedDirection><Source>ReferenceFrame</Source><SourceDirection>+X</SourceDirection><FeatureName></FeatureName></SecondaryAxis></Value></Frame><Frame><Id>Frame2</Id><Value><Name>F2</Name><Origin><Source>GeometricFeature</Source><FeatureName>point 1103</FeatureName></Origin><PrimaryAxis><DefinedDirection>+Z</DefinedDirection><Source>ReferenceFrame</Source><SourceDirection>+Z</SourceDirection><FeatureName></FeatureName></PrimaryAxis><SecondaryAxis><DefinedDirection>+X</DefinedDirection><Source>ReferenceFrame</Source><SourceDirection>+X</SourceDirection><FeatureName></FeatureName></SecondaryAxis></Value></Frame><Frame><Id>Frame3</Id><Value><Name>F3</Name><Origin><Source>GeometricFeature</Source><FeatureName>point 1083</FeatureName></Origin><PrimaryAxis><DefinedDirection>+Z</DefinedDirection><Source>ReferenceFrame</Source><SourceDirection>+Z</SourceDirection><FeatureName></FeatureName></PrimaryAxis><SecondaryAxis><DefinedDirection>+X</DefinedDirection><Source>ReferenceFrame</Source><SourceDirection>+X</SourceDirection><FeatureName></FeatureName></SecondaryAxis></Value></Frame><Frame><Id>Frame4</Id><Value><Name>F4</Name><Origin><Source>GeometricFeature</Source><FeatureName>point 1086</FeatureName></Origin><PrimaryAxis><DefinedDirection>+Z</DefinedDirection><Source>ReferenceFrame</Source><SourceDirection>+Z</SourceDirection><FeatureName></FeatureName></PrimaryAxis><SecondaryAxis><DefinedDirection>+X</DefinedDirection><Source>ReferenceFrame</Source><SourceDirection>+X</SourceDirection><FeatureName></FeatureName></SecondaryAxis></Value></Frame></Frames>  GraphicType=FromGeometry  MarkerShape=Sphere  MarkerSize=10  GraphicVisPropType=SimpleVisualProperties  GraphicDiffuseColor=smiData.Solid(10).color  GraphicSpecularColor=[0.5 0.5 0.5 1.0]  GraphicAmbientColor=[0.15 0.15 0.15 1.0]  GraphicEmissiveColor=[0.0 0.0 0.0 1.0]  GraphicShininess=75  GraphicOpacity=smiData.Solid(10).opacity  GeometryShape=FromFile  RectangleSize=[1 1]  RectangleSizeUnits=m  BrickDimensions=[1 1 1]  BrickDimensionUnits=m  CylinderRadius=1  CylinderRadiusUnits=m  CylinderLength=1  CylinderLengthUnits=m  SphereRadius=1  SphereRadiusUnits=m  EllipsoidRadii=[1 1 1]  EllipsoidRadiiUnits=m  ExtrusionCrossSection=[1 1; -1 1; -1 -1; 1 -1]  ExtrusionCrossSectionUnits=m  ExtrusionLength=1  ExtrusionLengthUnits=m  PolygonNumSides=3  PolygonOuterRadius=1  PolygonOuterRadiusUnits=m  ExtGeomFileType=STEP  ExtGeomFileName=left_ankle_twist_part_Default_sldprt.STEP  ExtGeomFileUnits=m  RevolutionCrossSection=[1 1; 1 -1; 2 -1; 2 1]  RevolutionCrossSectionUnits=m  RevolutionExtent=Full  RevolutionAngle=180  RevolutionAngleUnits=deg
  Sphere to Plane Force{,1..3} (4 alike) : Contact_Forces_Lib/3D/Sphere to Plane Force  sphere_rad=0.0001  plane_lenx=25  plane_leny=3  plane_depth=0.025/2  force_law=Linear  k_contact=1e4  b_contact=1e2  pen_full_damp_F=1e-4  pen_exponent=1  custom_param_1=1  custom_param_2=1  friction_law=Stick-Slip Continuous  mu_kinetic=0.5  mu_static=0.7  v_thr=0.001  vis_on=off  vis_opc_en=0  vis_len_plaBz=0.005  vis_clr=[0.9 0.2 0.2]  vis_opc=0.7
  Transform : sm_lib/Frames and Transforms/Rigid Transform  TranslationMethod=Cartesian  TranslationStandardOffset=0  TranslationLengthUnit=mm  TranslationStandardAxis=+Z  TranslationCartesianOffset=smiData.RigidTransform(12).translation  TranslationROffset=0  TranslationROffsetUnits=m  TranslationZOffset=0  TranslationZOffsetUnits=m  TranslationThetaOffset=0  TranslationThetaOffsetUnits=deg  RotationMethod=ArbitraryAxis  RotationAngleUnits=rad  RotationStandardAxis=+Z  RotationAngle=smiData.RigidTransform(12).angle  RotationArbitraryAxis=smiData.RigidTransform(12).axis  FollAlignAxisA=+X  BaseAlignAxisA=+Y  FollAlignAxisB=+Y  BaseAlignAxisB=+Z  RotationSequenceAxes=FollowerAxes  RotationSequence=XYX  RotationSequenceAngles=[0 0 0]  RotationSequenceAnglesUnits=deg  RotationMatrix=[1 0 0; 0 1 0; 0 0 1]
  left_abduction_RIGID : Subsystem
  left_ankle_RIGID : Subsystem
  left_flextion_RIGID : Subsystem
  left_knee_RIGID : Subsystem
  left_rotation_RIGID : Subsystem
  H : PMIOPort  Side=Left
  G : PMIOPort  Port=2  Side=Right
  meas : Outport
  wires:
  Demux/2 -> Simulink-PS Converter2/1
  Demux/5 -> Simulink-PS Converter5/1
  Demux/1 -> Simulink-PS Converter3/1
  qRef/1 -> Demux/1
  Demux/3 -> Simulink-PS Converter/1
  Demux/4 -> Simulink-PS Converter1/1
  Demux/6 -> Simulink-PS Converter4/1
  Knee Meas/1(meas) -> All measurements/5(knee)
  All measurements/1(meas) -> meas/1
  Ankle Meas/1(meas) -> All measurements/4(ankle)
  Abduction Meas/1(meas) -> All measurements/7(abduction)
  Contact Force Logging/2 -> All measurements/2(Ff)
  Ankle Twist Meas/1(meas) -> All measurements/3(ankle_twist)
  Hip Meas/1(meas) -> All measurements/6(hip)
  Rotation Meas/1(meas) -> All measurements/8(rotation)
  Contact Force Logging/1 -> All measurements/1(Fn)
  Sphere to Plane Force/1 -> Contact Force Logging/1
  Sphere to Plane Force1/1 -> Contact Force Logging/2
  Sphere to Plane Force2/1 -> Contact Force Logging/3
  Sphere to Plane Force3/1 -> Contact Force Logging/4
  connections:
  Knee_joint/LConn1 -- left_flextion_RIGID/RConn1
  Ankle_joint/RConn1 -- left_knee_RIGID/LConn1
  Ankle_joint/LConn1 -- left_ankle_RIGID/RConn1
  H/RConn1 -- Left_Rotation_Joint/LConn1
  Left_Ankle_Twist_Joint/LConn1 -- left_ankle_RIGID/LConn1
  Left_Rotation_Joint/RConn1 -- left_rotation_RIGID/RConn1
  Hip_Joint/LConn1 -- left_abduction_RIGID/RConn1
  Knee_joint/RConn1 -- left_knee_RIGID/RConn1
  Left_Abduction_Joint/LConn1 -- left_abduction_RIGID/LConn1
  Hip_Joint/RConn1 -- left_flextion_RIGID/LConn1
  Left_Abduction_Joint/RConn1 -- left_rotation_RIGID/LConn1
  Transform/RConn1 -- Left_Ankle_Twist_Joint/RConn1
  Simulink-PS Converter4/RConn1 -- Left_Rotation_Joint/LConn2
  Simulink-PS Converter2/RConn1 -- Ankle_joint/LConn2
  Left_Ankle_Twist_Joint/LConn2 -- Simulink-PS Converter3/RConn1
  Simulink-PS Converter5/RConn1 -- Left_Abduction_Joint/LConn2
  Simulink-PS Converter1/RConn1 -- Hip_Joint/LConn2
  Knee_joint/LConn2 -- Simulink-PS Converter/RConn1
  Sphere to Plane Force3/RConn1 -- Sphere to Plane Force2/RConn1 -- Sphere to Plane Force/RConn1 -- Sphere to Plane Force1/RConn1 -- G/RConn1
  Solid/LConn1 -- Sphere to Plane Force/LConn1
  Solid/LConn2 -- Sphere to Plane Force2/LConn1
  Solid/RConn2 -- Sphere to Plane Force3/LConn1
  Solid/LConn3 -- Sphere to Plane Force1/LConn1
  Solid/RConn1 -- Transform/LConn1
  Left_Ankle_Twist_Joint/RConn2 -- Ankle Twist Meas/LConn1
  Left_Ankle_Twist_Joint/RConn3 -- Ankle Twist Meas/LConn2
  Left_Ankle_Twist_Joint/RConn4 -- Ankle Twist Meas/LConn3
  Ankle_joint/RConn2 -- Ankle Meas/LConn1
  Ankle_joint/RConn3 -- Ankle Meas/LConn2
  Ankle_joint/RConn4 -- Ankle Meas/LConn3
  Knee_joint/RConn2 -- Knee Meas/LConn1
  Knee_joint/RConn3 -- Knee Meas/LConn2
  Knee_joint/RConn4 -- Knee Meas/LConn3
  Hip_Joint/RConn2 -- Hip Meas/LConn1
  Hip_Joint/RConn3 -- Hip Meas/LConn2
  Hip_Joint/RConn4 -- Hip Meas/LConn3
  Left_Abduction_Joint/RConn2 -- Abduction Meas/LConn1
  Left_Abduction_Joint/RConn3 -- Abduction Meas/LConn2
  Left_Abduction_Joint/RConn4 -- Abduction Meas/LConn3
  Left_Rotation_Joint/RConn2 -- Rotation Meas/LConn1
  Left_Rotation_Joint/RConn3 -- Rotation Meas/LConn2
  Left_Rotation_Joint/RConn4 -- Rotation Meas/LConn3

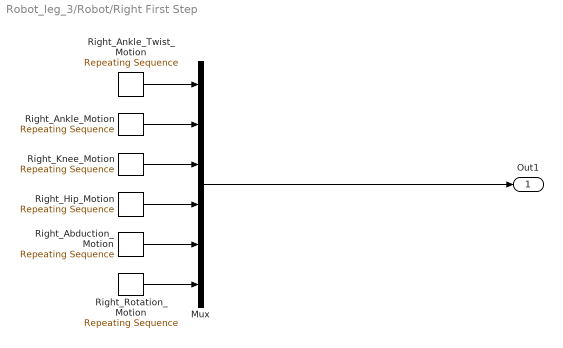
== system Robot_leg_3/Robot/Right First Step ==
  Mux : Mux  Inputs=6
  Right_Abduction_Motion : simulink/Sources/Repeating Sequence  rep_seq_t=time  rep_seq_y=right_theta_first_5
  Right_Ankle_Motion : simulink/Sources/Repeating Sequence  rep_seq_t=time  rep_seq_y=right_theta_first_3
  Right_Ankle_Twist_Motion : simulink/Sources/Repeating Sequence  rep_seq_t=time  rep_seq_y=right_theta_first_4
  Right_Hip_Motion : simulink/Sources/Repeating Sequence  rep_seq_t=time  rep_seq_y=right_theta_first_1
  Right_Knee_Motion : simulink/Sources/Repeating Sequence  rep_seq_t=time  rep_seq_y=right_theta_first_2
  Right_Rotation_Motion : simulink/Sources/Repeating Sequence  rep_seq_t=time_first  rep_seq_y=right_theta_first_6
  Out1 : Outport
  wires:
  Mux/1 -> Out1/1
  Right_Ankle_Motion/1 -> Mux/2
  Right_Ankle_Twist_Motion/1 -> Mux/1
  Right_Knee_Motion/1 -> Mux/3
  Right_Rotation_Motion/1 -> Mux/6
  Right_Abduction_Motion/1 -> Mux/5
  Right_Hip_Motion/1 -> Mux/4

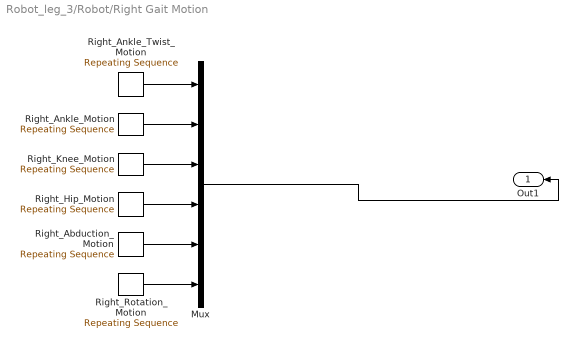
== system Robot_leg_3/Robot/Right Gait Motion ==
  Mux : Mux  Inputs=6
  Right_Abduction_Motion : simulink/Sources/Repeating Sequence  rep_seq_t=time  rep_seq_y=right_theta_5
  Right_Ankle_Motion : simulink/Sources/Repeating Sequence  rep_seq_t=time  rep_seq_y=right_theta_3
  Right_Ankle_Twist_Motion : simulink/Sources/Repeating Sequence  rep_seq_t=time  rep_seq_y=right_theta_4
  Right_Hip_Motion : simulink/Sources/Repeating Sequence  rep_seq_t=time  rep_seq_y=right_theta_1
  Right_Knee_Motion : simulink/Sources/Repeating Sequence  rep_seq_t=time  rep_seq_y=right_theta_2
  Right_Rotation_Motion : simulink/Sources/Repeating Sequence  rep_seq_t=time  rep_seq_y=right_theta_6
  Out1 : Outport
  wires:
  Mux/1 -> Out1/1
  Right_Ankle_Motion/1 -> Mux/2
  Right_Ankle_Twist_Motion/1 -> Mux/1
  Right_Knee_Motion/1 -> Mux/3
  Right_Rotation_Motion/1 -> Mux/6
  Right_Abduction_Motion/1 -> Mux/5
  Right_Hip_Motion/1 -> Mux/4

== system Robot_leg_3/Robot/Right Gait Pos ==
  Mux : Mux  Inputs=6
  Right_Abduction_Motion : simulink/Sources/Repeating Sequence  rep_seq_t=time  rep_seq_y=right_theta_pos_5
  Right_Ankle_Motion : simulink/Sources/Repeating Sequence  rep_seq_t=time  rep_seq_y=right_theta_pos_3
  Right_Ankle_Twist_Motion : simulink/Sources/Repeating Sequence  rep_seq_t=time  rep_seq_y=right_theta_pos_4
  Right_Hip_Motion : simulink/Sources/Repeating Sequence  rep_seq_t=time  rep_seq_y=right_theta_pos_1
  Right_Knee_Motion : simulink/Sources/Repeating Sequence  rep_seq_t=time  rep_seq_y=right_theta_pos_2
  Right_Rotation_Motion : simulink/Sources/Repeating Sequence  rep_seq_t=time  rep_seq_y=right_theta_pos_6
  Out1 : Outport
  wires:
  Mux/1 -> Out1/1
  Right_Rotation_Motion/1 -> Mux/6
  Right_Hip_Motion/1 -> Mux/4
  Right_Ankle_Twist_Motion/1 -> Mux/1
  Right_Knee_Motion/1 -> Mux/3
  Right_Abduction_Motion/1 -> Mux/5
  Right_Ankle_Motion/1 -> Mux/2

== system Robot_leg_3/Robot/Right Still ==
  Mux : Mux  Inputs=6
  Right_Abduction_Motion : simulink/Sources/Repeating Sequence  rep_seq_t=time  rep_seq_y=right_theta_init_5
  Right_Ankle_Motion : simulink/Sources/Repeating Sequence  rep_seq_t=time  rep_seq_y=right_theta_init_3
  Right_Ankle_Twist_Motion : simulink/Sources/Repeating Sequence  rep_seq_t=time  rep_seq_y=right_theta_init_4
  Right_Hip_Motion : simulink/Sources/Repeating Sequence  rep_seq_t=time  rep_seq_y=right_theta_init_1
  Right_Knee_Motion : simulink/Sources/Repeating Sequence  rep_seq_t=time  rep_seq_y=right_theta_init_2
  Right_Rotation_Motion : simulink/Sources/Repeating Sequence  rep_seq_t=time  rep_seq_y=right_theta_init_6
  Out1 : Outport
  wires:
  Mux/1 -> Out1/1
  Right_Rotation_Motion/1 -> Mux/6
  Right_Hip_Motion/1 -> Mux/4
  Right_Ankle_Twist_Motion/1 -> Mux/1
  Right_Knee_Motion/1 -> Mux/3
  Right_Abduction_Motion/1 -> Mux/5
  Right_Ankle_Motion/1 -> Mux/2
